simulink model "prvi"  (R2017b)
settings: Solver=ode15s  StartTime=0.0  StopTime=10.0  RelTol=1e-3
values from neighbouring files (symbols this model uses):
  Kt = 0.02    [matematicki_model_motora.m]
  L = 0.2    [matematicki_model_motora.m]
  R = 1    [matematicki_model_motora.m]
undefined symbols (not defined in the file or in its folder): iL, Km
settings Model: Creator=DT User  LastModifiedBy=DT User

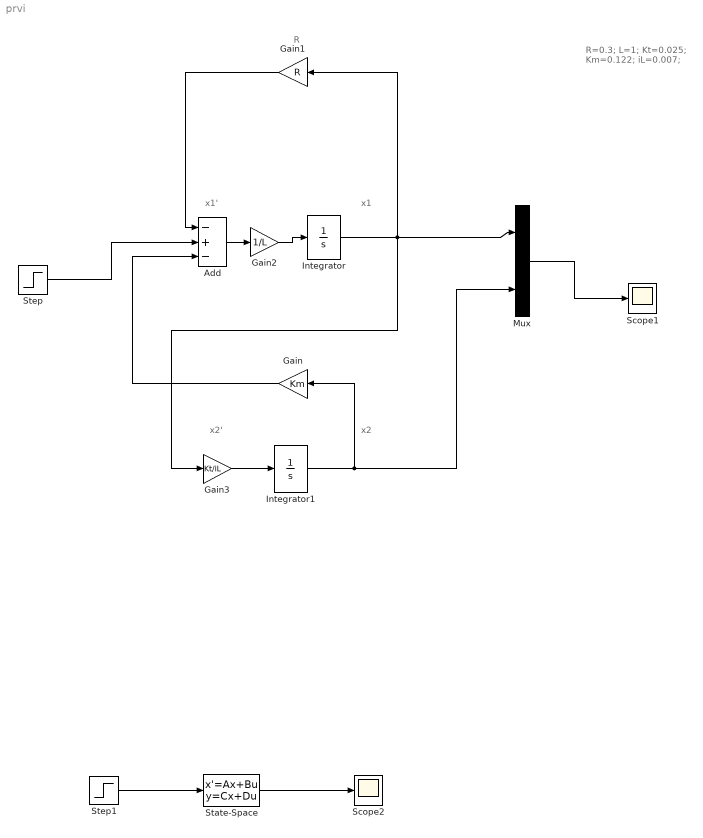
== system prvi ==
  note: R=0.3;
      | L=1;
      | Kt=0.025;
      | Km=0.122;
      | iL=0.007;
  note: R
  note: x1'
  note: x1
  note: x2
  note: x2'
  Add : Sum  Inputs=-+-
  Gain : Gain  Gain=Km
  Gain1 : Gain  Gain=R
  Gain2 : Gain  Gain=1/L
  Gain3 : Gain  Gain=Kt/iL
  Integrator : Integrator
  Integrator1 : Integrator
  Mux : Mux  Inputs=2
  Scope1 : Scope
  Scope2 : Scope
  State-Space : StateSpace  A=[-0.3/1 -0.122/1 ;0.025/0.007 0]  B=[1/1; 0]  C=[1 0 ; 0 1]  D=[0;0]  InitialCondition=0
  Step : Step  Time=0  SampleTime=0
  Step1 : Step  Time=0  SampleTime=0
  wires:
  Step/1 -> Add/2
  Mux/1 -> Scope1/1
  Integrator/1 -> Gain1/1, Mux/1, Gain3/1
  Integrator1/1 -> Gain/1, Mux/2
  Gain1/1 -> Add/1
  Add/1 -> Gain2/1
  Gain2/1 -> Integrator/1
  Gain/1 -> Add/3
  Gain3/1 -> Integrator1/1
  Step1/1 -> State-Space/1
  State-Space/1 -> Scope2/1
